simulink model "surface"  (R2016b)
settings: Solver=VariableStepAuto  StartTime=0.0  StopTime=10.0  RelTol=1e-3
settings Model: Creator=charAn  LastModifiedBy=charAn

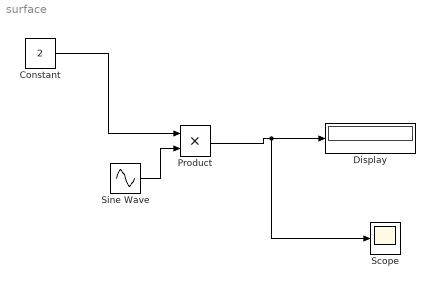
== system surface ==
  Constant : Constant  Value=2
  Display : Display
  Product : Product
  Scope : Scope
  Sine Wave : Sin  Phase=0.6981  SampleTime=0
  wires:
  Constant/1 -> Product/1
  Product/1 -> Scope/1, Display/1
  Sine Wave/1 -> Product/2
